simulink model "Path_Planning_Subsystem_Simulink"  (R2021a)
settings: Solver=VariableStepAuto  StartTime=0.0  StopTime=5  RelTol=1e-3
settings Model: Creator=WU  LastModifiedBy=WU

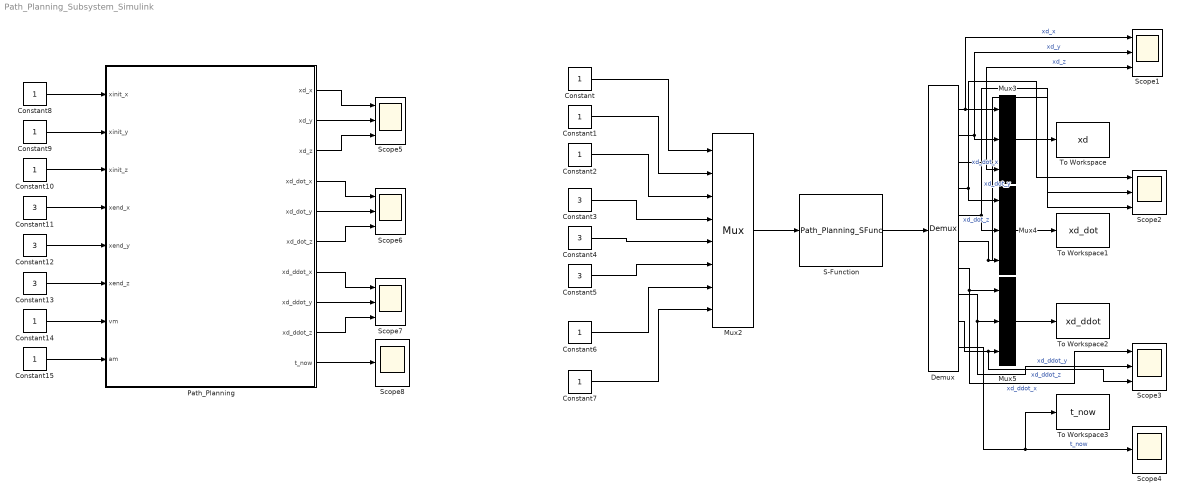
== system Path_Planning_Subsystem_Simulink ==
  Constant : Constant  VectorParams1D=off
  Constant{1..2,6..7,9..10,14..15} (8 alike) : Constant
  Constant{3..5,11..13} (6 alike) : Constant  Value=3
  Constant8 : Constant  VectorParams1D=off
  Demux : Demux  Outputs=10
      settings: DisplayOption=none
  Mux2 : Mux  Inputs=8
  Mux3 : Mux  Inputs=3
  Mux4 : Mux  Inputs=3
  Mux5 : Mux  Inputs=3
  Path_Planning : Subsystem
  S-Function : S-Function  FunctionName=Path_Planning_SFunc  SFunctionDeploymentMode=off  EnableBusSupport=off
  Scope{1..3,5..7} (6 alike) : Scope  NumInputPorts=3
  Scope4 : Scope
  Scope8 : Scope
  To Workspace : ToWorkspace  VariableName=xd  SampleTime=-1
  To Workspace1 : ToWorkspace  VariableName=xd_dot  SampleTime=-1
  To Workspace2 : ToWorkspace  VariableName=xd_ddot  SampleTime=-1
  To Workspace3 : ToWorkspace  VariableName=t_now  SampleTime=-1
  wires:
  Constant/1 -> Mux2/1
  Constant2/1 -> Mux2/3
  Constant3/1 -> Mux2/4
  Constant4/1 -> Mux2/5
  Constant5/1 -> Mux2/6
  Mux2/1 -> S-Function/1
  S-Function/1 -> Demux/1
  Demux/1 -> Scope1/1, Mux3/1  "xd_x"
  Demux/2 -> Mux3/2, Scope1/2  "xd_y"
  Demux/3 -> Mux3/3, Scope1/3  "xd_z"
  Mux3/1 -> To Workspace/1
  Demux/4 -> Mux4/1, Scope2/1  "xd_dot_x"
  Demux/6 -> Scope2/3, Mux4/3  "xd_dot_z"
  Demux/5 -> Mux4/2, Scope2/2  "xd_dot_y"
  Mux4/1 -> To Workspace1/1
  Demux/7 -> Scope3/1, Mux5/1  "xd_ddot_x"
  Demux/8 -> Scope3/2, Mux5/2  "xd_ddot_y"
  Demux/9 -> Scope3/3, Mux5/3  "xd_ddot_z"
  Mux5/1 -> To Workspace2/1
  Constant1/1 -> Mux2/2
  Constant6/1 -> Mux2/7
  Constant7/1 -> Mux2/8
  Demux/10 -> To Workspace3/1, Scope4/1  "t_now"
  Constant8/1 -> Path_Planning/1(xinit_x)
  Constant9/1 -> Path_Planning/2(xinit_y)
  Constant10/1 -> Path_Planning/3(xinit_z)
  Constant11/1 -> Path_Planning/4(xend_x)
  Constant12/1 -> Path_Planning/5(xend_y)
  Constant13/1 -> Path_Planning/6(xend_z)
  Constant14/1 -> Path_Planning/7(vm)
  Constant15/1 -> Path_Planning/8(am)
  Path_Planning/1(xd_x) -> Scope5/1
  Path_Planning/2(xd_y) -> Scope5/2
  Path_Planning/3(xd_z) -> Scope5/3
  Path_Planning/4(xd_dot_x) -> Scope6/1
  Path_Planning/5(xd_dot_y) -> Scope6/2
  Path_Planning/6(xd_dot_z) -> Scope6/3
  Path_Planning/8(xd_ddot_y) -> Scope7/2
  Path_Planning/7(xd_ddot_x) -> Scope7/1
  Path_Planning/9(xd_ddot_z) -> Scope7/3
  Path_Planning/10(t_now) -> Scope8/1

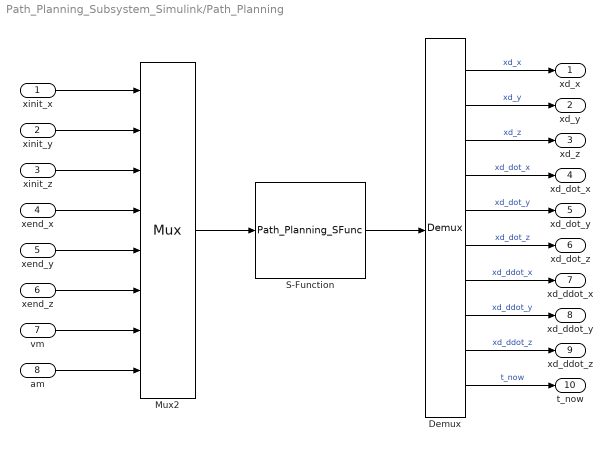
== system Path_Planning_Subsystem_Simulink/Path_Planning ==
  xinit_x : Inport
  xinit_y : Inport  Port=2
  xinit_z : Inport  Port=3
  xend_x : Inport  Port=4
  xend_y : Inport  Port=5
  xend_z : Inport  Port=6
  vm : Inport  Port=7
  am : Inport  Port=8
  Demux : Demux  Outputs=10
      settings: DisplayOption=none
  Mux2 : Mux  Inputs=8
  S-Function : S-Function  FunctionName=Path_Planning_SFunc  SFunctionDeploymentMode=off  EnableBusSupport=off
  xd_x : Outport
  xd_y : Outport  Port=2
  xd_z : Outport  Port=3
  xd_dot_x : Outport  Port=4
  xd_dot_y : Outport  Port=5
  xd_dot_z : Outport  Port=6
  xd_ddot_x : Outport  Port=7
  xd_ddot_y : Outport  Port=8
  xd_ddot_z : Outport  Port=9
  t_now : Outport  Port=10
  wires:
  Demux/7 -> xd_ddot_x/1  "xd_ddot_x"
  vm/1 -> Mux2/7
  xinit_y/1 -> Mux2/2
  Demux/1 -> xd_x/1  "xd_x"
  Demux/4 -> xd_dot_x/1  "xd_dot_x"
  Demux/5 -> xd_dot_y/1  "xd_dot_y"
  Demux/9 -> xd_ddot_z/1  "xd_ddot_z"
  Demux/8 -> xd_ddot_y/1  "xd_ddot_y"
  Demux/3 -> xd_z/1  "xd_z"
  Demux/6 -> xd_dot_z/1  "xd_dot_z"
  Demux/2 -> xd_y/1  "xd_y"
  xend_y/1 -> Mux2/5
  Mux2/1 -> S-Function/1
  S-Function/1 -> Demux/1
  xend_z/1 -> Mux2/6
  xend_x/1 -> Mux2/4
  xinit_z/1 -> Mux2/3
  xinit_x/1 -> Mux2/1
  am/1 -> Mux2/8
  Demux/10 -> t_now/1  "t_now"
